simulink model "P3_Model_Final_V2"  (R2023b)
settings: Solver=VariableStepAuto  StartTime=0.0  StopTime=10.0  RelTol=1e-3
values from neighbouring files (symbols this model uses):
  DriveData = DriveData_urban    [Project3_RunSim_Final.m]
undefined symbols (not defined in the file or in its folder): batData, C0, C1, C2, carData, Iw, M, motorData, mph2mps, r, rps2rpm, Time
libraries: slpidlib x1
settings Model: Creator=jessi  LastModifiedBy=jessi

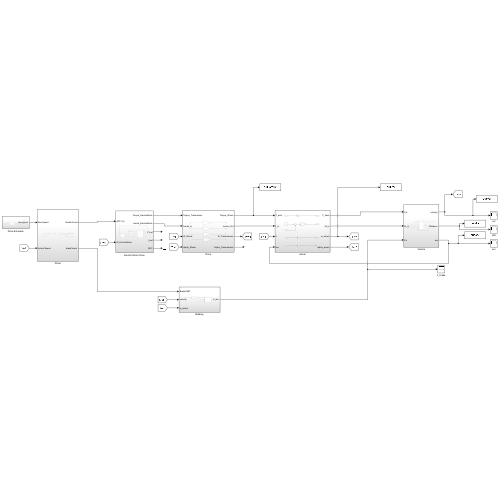
[thumbnail: Simulink's stored preview of the top-level diagram]
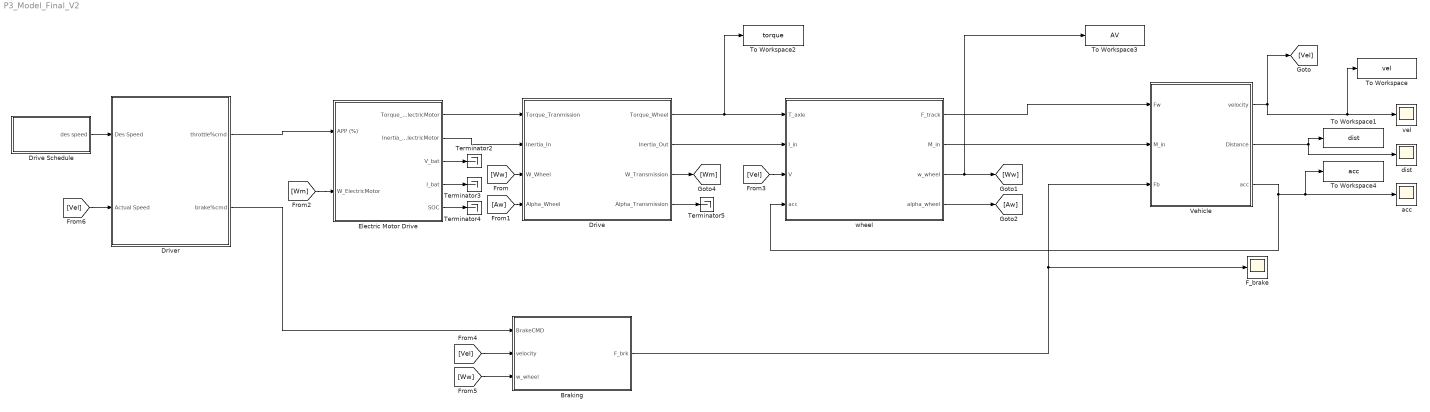
== system P3_Model_Final_V2 ==
  Braking : Subsystem
  Drive : Subsystem
  Drive Schedule : Subsystem
  "Driver " : Subsystem
  Electric Motor Drive : Subsystem
  F_brake : Scope
  Terminator{2..5} (4 alike) : Terminator
  To Workspace : ToWorkspace  VariableName=vel  SaveFormat=Timeseries  SampleTime=-1
  To Workspace1 : ToWorkspace  VariableName=dist  SaveFormat=Timeseries  SampleTime=-1
  To Workspace2 : ToWorkspace  VariableName=torque  SaveFormat=Timeseries  SampleTime=-1
  To Workspace3 : ToWorkspace  VariableName=AV  SaveFormat=Timeseries  SampleTime=-1
  To Workspace4 : ToWorkspace  VariableName=acc  SaveFormat=Timeseries  SampleTime=-1
  Vehicle : Subsystem
  acc : Scope
  dist : Scope
  vel : Scope
  "wheel " : Subsystem
  wires:
  [Ww] -> Braking/3(w_wheel)
  [Vel] -> Braking/2("velocity ")
  "wheel "/3(w_wheel) -> To Workspace3/1, [Ww]
  "wheel "/1(F_track) -> Vehicle/1("Fw ")
  [Wm] -> Electric Motor Drive/2(W_ElectricMotor)
  "wheel "/2(M_in) -> Vehicle/2("M_in ")
  [Ww] -> Drive/3(W_Wheel)
  Drive/1(Torque_Wheel) -> To Workspace2/1, "wheel "/1(T_axle)
  Drive/2(Inertia_Out) -> "wheel "/2(I_in)
  Electric Motor Drive/4(I_bat) -> Terminator3/1
  [Vel] -> "wheel "/3(V)
  Electric Motor Drive/5(SOC) -> Terminator4/1
  Electric Motor Drive/3(V_bat) -> Terminator2/1
  Vehicle/2("Distance ") -> dist/1, To Workspace1/1
  Braking/1("F_brk ") -> F_brake/1, Vehicle/3("Fb ")
  Drive/4(Alpha_Transmission) -> Terminator5/1
  Electric Motor Drive/2(Inertia_ElectricMotor) -> Drive/2(Inertia_In)
  Vehicle/3(acc) -> "wheel "/4(acc), To Workspace4/1, acc/1
  Vehicle/1("velocity ") -> To Workspace/1, vel/1, [Vel]
  Electric Motor Drive/1(Torque_ElectricMotor) -> Drive/1(Torque_Tranmission)
  "wheel "/4(alpha_wheel) -> [Aw]
  [Aw] -> Drive/4(Alpha_Wheel)
  Drive/3(W_Transmission) -> [Wm]
  Drive Schedule/1("des speed ") -> "Driver "/1("Des Speed ")
  [Vel] -> "Driver "/2(Actual Speed)
  "Driver "/1(throttle%cmd) -> Electric Motor Drive/1(APP (%))
  "Driver "/2("brake%cmd ") -> Braking/1("BrakeCMD ")

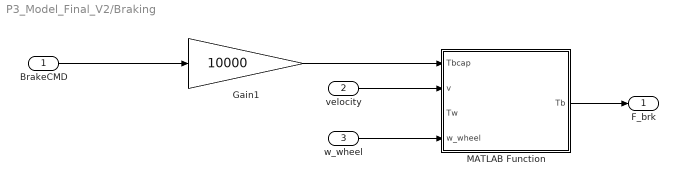
== system P3_Model_Final_V2/Braking ==
  "BrakeCMD " : Inport
  "velocity " : Inport  Port=2
  w_wheel : Inport  Port=3
  Gain1 : Gain  Gain=10000
  MATLAB Function : MATLAB Function  TreatAsAtomicUnit=on
  "F_brk " : Outport  VectorParamsAs1DForOutWhenUnconnected=off
  wires:
  "BrakeCMD "/1 -> Gain1/1
  Gain1/1 -> MATLAB Function/1(Tbcap)
  MATLAB Function/1(Tb) -> "F_brk "/1
  "velocity "/1 -> MATLAB Function/2(v)
  w_wheel/1 -> MATLAB Function/4(w_wheel)

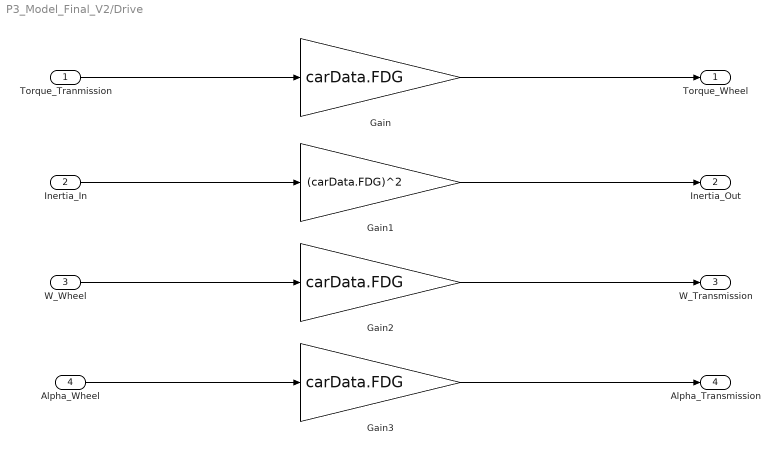
== system P3_Model_Final_V2/Drive ==
  Torque_Tranmission : Inport
  Inertia_In : Inport  Port=2
  W_Wheel : Inport  Port=3
  Alpha_Wheel : Inport  Port=4
  Gain : Gain  Gain=carData.FDG
  Gain1 : Gain  Gain=(carData.FDG)^2
  Gain2 : Gain  Gain=carData.FDG
  Gain3 : Gain  Gain=carData.FDG
  Torque_Wheel : Outport
  Inertia_Out : Outport  Port=2
  W_Transmission : Outport  Port=3
  Alpha_Transmission : Outport  Port=4
  wires:
  Torque_Tranmission/1 -> Gain/1
  Inertia_In/1 -> Gain1/1
  W_Wheel/1 -> Gain2/1
  Alpha_Wheel/1 -> Gain3/1
  Gain/1 -> Torque_Wheel/1
  Gain1/1 -> Inertia_Out/1
  Gain2/1 -> W_Transmission/1
  Gain3/1 -> Alpha_Transmission/1

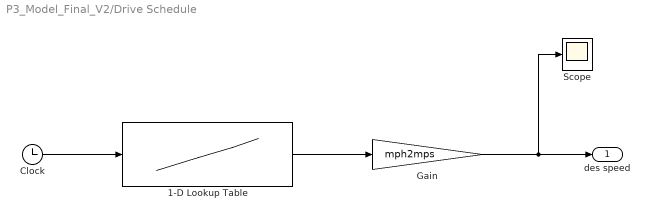
== system P3_Model_Final_V2/Drive Schedule ==
  1-D Lookup Table : Lookup_n-D  NumberOfTableDimensions=1  BreakpointsForDimension1=Time  Table=DriveData  InternalRulePriority=Speed  RndMeth=Simplest
  Clock : Clock
  Gain : Gain  Gain=mph2mps
  Scope : Scope
  "des speed " : Outport  VectorParamsAs1DForOutWhenUnconnected=off
  wires:
  Clock/1 -> 1-D Lookup Table/1
  1-D Lookup Table/1 -> Gain/1
  Gain/1 -> "des speed "/1, Scope/1

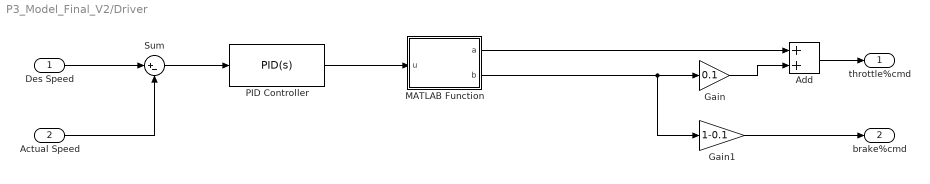
== system P3_Model_Final_V2/Driver  ==
  "Des Speed " : Inport
  Actual Speed : Inport  Port=2
  Add : Sum
  Gain : Gain  Gain=0.1
  Gain1 : Gain  Gain=1-0.1
  MATLAB Function : MATLAB Function  TreatAsAtomicUnit=on
  PID Controller : slpidlib/PID Controller  Controller=PID  Form=Parallel  TimeDomain=Continuous-time  UseExternalTs=off  SampleTime=-1  IntegratorMethod=Forward Euler  FilterMethod=Forward Euler  ControllerParametersSource=internal  P=0.55  I=0  UseKiTs=off  D=0  N=100  UseFilter=on  TunerSelectOption=Transfer Function Based (PID Tuner App)  InitialConditionSource=internal  InitialConditionForIntegrator=0  InitialConditionForFilter=0  DifferentiatorICPrevScaledInput=0  ExternalReset=none  TrackingMode=off  Kt=1  LimitOutput=on  SatLimitsSource=internal  UpperSaturationLimit=1  LowerSaturationLimit=-1  LinearizeAsGain=off  AntiWindupMode=none  Kb=1  LimitIntegrator=off  UpperIntegratorSaturationLimit=inf  LowerIntegratorSaturationLimit=-inf  POutMin=[]  POutMax=[]  IOutMin=[]  IOutMax=[]  DOutMin=[]  DOutMax=[]  NOutMin=[]  NOutMax=[]  SumOutMin=[]  SumOutMax=[]  SaturationOutMin=[]  SaturationOutMax=[]  PParamMin=[]  PParamMax=[]  IParamMin=[]  IParamMax=[]  DParamMin=[]  DParamMax=[]  NParamMin=[]  NParamMax=[]  KbParamMin=[]  KbParamMax=[]  KtParamMin=[]  KtParamMax=[]  KbOutMin=[]  KbOutMax=[]  KtOutMin=[]  KtOutMax=[]  IntegratorOutMin=[]  IntegratorOutMax=[]  FilterOutMin=[]  FilterOutMax=[]  SumI1OutMin=[]  SumI1OutMax=[]  SumI2OutMin=[]  SumI2OutMax=[]  SumI3OutMin=[]  SumI3OutMax=[]  SumI4OutMin=[]  SumI4OutMax=[]  SumDOutMin=[]  SumDOutMax=[]  DifferentiatorOutMin=[]  DifferentiatorOutMax=[]  FilterDiffOutCoefMin=[]  FilterDiffOutCoefMax=[]  ReciprocalOutMin=[]  ReciprocalOutMax=[]  SumDenOutMin=[]  SumDenOutMax=[]  SumNumOutMin=[]  SumNumOutMax=[]  DivideOutMin=[]  DivideOutMax=[]  UdiffTsProdOutMin=[]  UdiffTsProdOutMax=[]  NTsProdOutMin=[]  NTsProdOutMax=[]  UintegralTsProdOutMin=[]  UintegralTsProdOutMax=[]  UngainTsProdOutMin=[]  UngainTsProdOutMax=[]  ClampingZeroOutDataTypeStr=Inherit: Inherit via back propagation  ClampingZeroOutMin=[]  ClampingZeroOutMax=[]  FilterDenConstantOutDataTypeStr=Inherit: Inherit via back propagation  FilterDenConstantOutMin=[]  FilterDenConstantOutMax=[]  PCopyOutDataTypeStr=Inherit: Inherit via back propagation  PCopyOutMin=[]  PCopyOutMax=[]  NCopyOutDataTypeStr=Inherit: Inherit via back propagation  NCopyOutMin=[]  NCopyOutMax=[]  IntegratorContinuousStateAttributes=''  IntegratorStateMustResolveToSignalObject=off  IntegratorRTWStateStorageClass=Auto  FilterContinuousStateAttributes=''  FilterStateMustResolveToSignalObject=off  FilterRTWStateStorageClass=Auto  ParallelPVariant=InternalParameters  IdealPVariant=Disabled  IVariant=InternalParameters  DVariant=InternalParameters  IntegratorVariant=Continuous  SatVariant=Enabled  AWVariant=Passthrough  PCopyVariant=Disabled  TRVariant=Disabled  FdbkBlocksVariant=Forward  IdealPFdbkVariant=Disabled  SatFdbkVariant=Disabled  DerivativeFilterVariant=ContFilter  NVariant=InternalParameters  NCopyVariant=Disabled  FilterICVariant=InternalICsFilter  IntegratorICVariant=InternalICs  ExternalResetVariant=Disabled  TRSumVariant=Passthrough  SumFdbkVariant=Disabled  SumVariant=Sum_PID  TsampFilterVariant=InternalTs  TsampNgainVariant=Passthrough  TsampIntegralVariant=Disabled_SignalSpec  ExternalSaturationOutDataTypeStr=Inherit: Same as second input
  Sum : Sum  Inputs=|+-
  throttle%cmd : Outport
  "brake%cmd " : Outport  Port=2
  wires:
  MATLAB Function/1(a) -> Add/1
  Gain/1 -> Add/2
  Add/1 -> throttle%cmd/1
  Gain1/1 -> "brake%cmd "/1
  MATLAB Function/2(b) -> Gain1/1, Gain/1
  Sum/1 -> PID Controller/1
  PID Controller/1 -> MATLAB Function/1(u)
  "Des Speed "/1 -> Sum/1
  Actual Speed/1 -> Sum/2

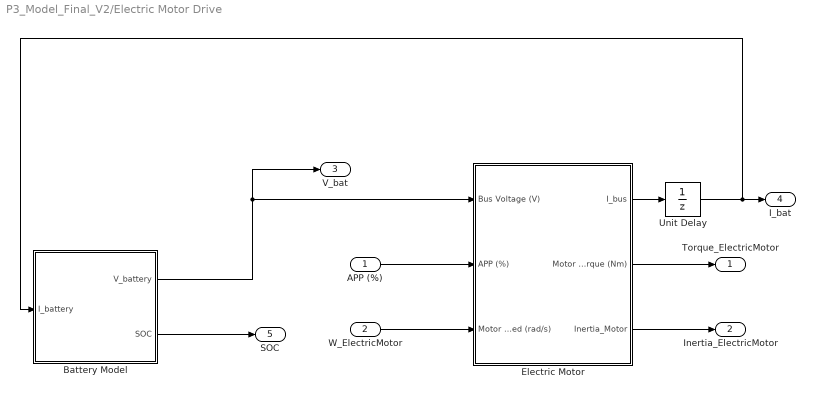
== system P3_Model_Final_V2/Electric Motor Drive ==
  APP (%) : Inport
  W_ElectricMotor : Inport  Port=2
  Battery Model : Subsystem  TreatAsAtomicUnit=on
  Electric Motor : Subsystem  TreatAsAtomicUnit=on
  Unit Delay : UnitDelay  SampleTime=-1  HasFrameUpgradeWarning=on
  Torque_ElectricMotor : Outport
  Inertia_ElectricMotor : Outport  Port=2
  V_bat : Outport  Port=3
  I_bat : Outport  Port=4
  SOC : Outport  Port=5
  wires:
  Electric Motor/2(Motor Torque (Nm)) -> Torque_ElectricMotor/1
  Battery Model/2(SOC) -> SOC/1
  Electric Motor/3(Inertia_Motor) -> Inertia_ElectricMotor/1
  W_ElectricMotor/1 -> Electric Motor/3(Motor Speed (rad/s))
  Electric Motor/1(I_bus) -> Unit Delay/1
  APP (%)/1 -> Electric Motor/2(APP (%))
  Battery Model/1(V_battery) -> Electric Motor/1(Bus Voltage (V)), V_bat/1
  Unit Delay/1 -> Battery Model/1(I_battery), I_bat/1

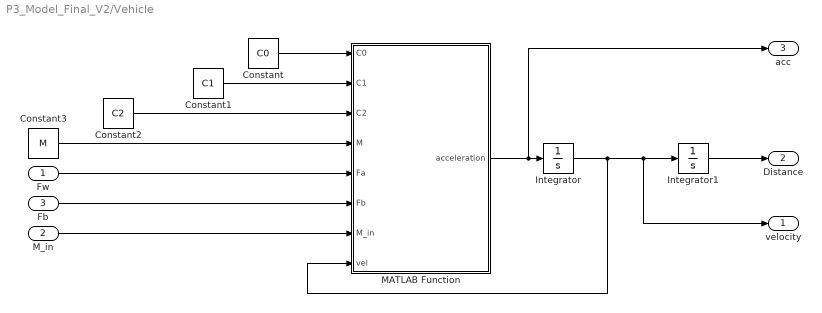
== system P3_Model_Final_V2/Vehicle ==
  "Fw " : Inport
  "M_in " : Inport  Port=2
  "Fb " : Inport  Port=3
  Constant : Constant  Value=C0
  Constant1 : Constant  Value=C1
  Constant2 : Constant  Value=C2
  Constant3 : Constant  Value=M
  Integrator : Integrator  LimitOutput=on  LowerSaturationLimit=0
  Integrator1 : Integrator
  MATLAB Function : MATLAB Function  TreatAsAtomicUnit=on
  "velocity " : Outport  VectorParamsAs1DForOutWhenUnconnected=off
  "Distance " : Outport  Port=2  VectorParamsAs1DForOutWhenUnconnected=off
  acc : Outport  Port=3
  wires:
  Constant1/1 -> MATLAB Function/2(C1)
  Constant/1 -> MATLAB Function/1(C0)
  MATLAB Function/1(acceleration) -> acc/1, Integrator/1
  Constant2/1 -> MATLAB Function/3(C2)
  Constant3/1 -> MATLAB Function/4(M)
  "Fw "/1 -> MATLAB Function/5(Fa)
  "Fb "/1 -> MATLAB Function/6(Fb)
  Integrator/1 -> MATLAB Function/8(vel), "velocity "/1, Integrator1/1
  Integrator1/1 -> "Distance "/1
  "M_in "/1 -> MATLAB Function/7(M_in)

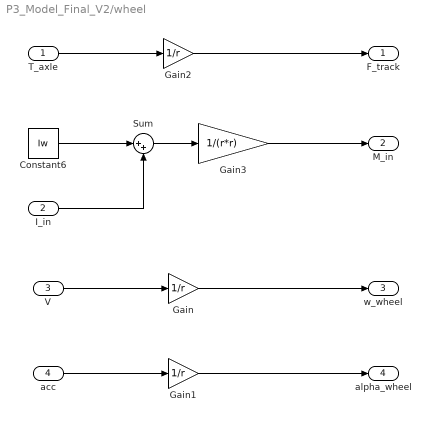
== system P3_Model_Final_V2/wheel  ==
  T_axle : Inport
  I_in : Inport  Port=2
  V : Inport  Port=3
  acc : Inport  Port=4
  Constant6 : Constant  Value=Iw
  Gain : Gain  Gain=1/r
  Gain1 : Gain  Gain=1/r
  Gain2 : Gain  Gain=1/r
  Gain3 : Gain  Gain=1/(r*r)
  Sum : Sum  Inputs=|++
  F_track : Outport
  M_in : Outport  Port=2
  w_wheel : Outport  Port=3
  alpha_wheel : Outport  Port=4
  wires:
  Gain/1 -> w_wheel/1
  V/1 -> Gain/1
  acc/1 -> Gain1/1
  Gain1/1 -> alpha_wheel/1
  T_axle/1 -> Gain2/1
  Gain2/1 -> F_track/1
  Gain3/1 -> M_in/1
  Constant6/1 -> Sum/1
  I_in/1 -> Sum/2
  Sum/1 -> Gain3/1

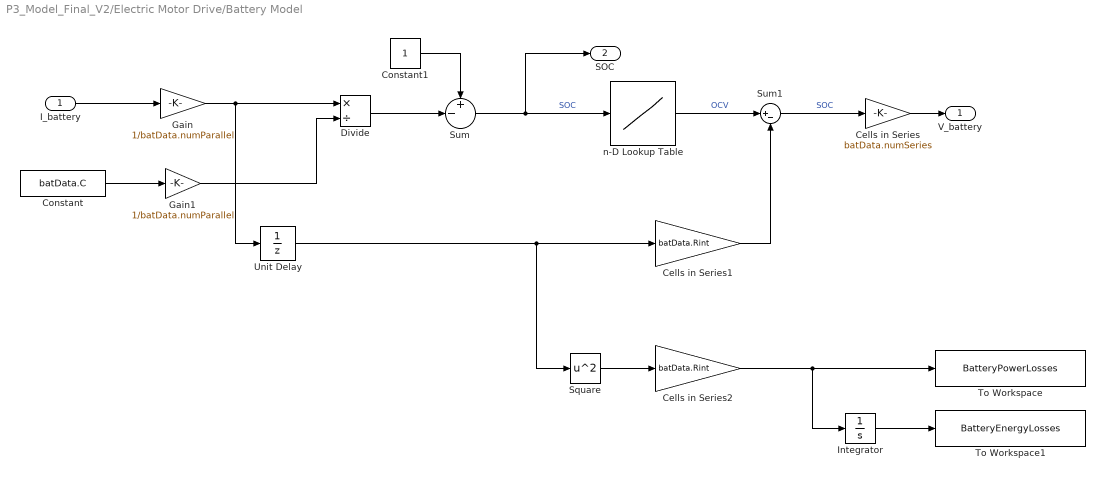
== system P3_Model_Final_V2/Electric Motor Drive/Battery Model ==
  I_battery : Inport
  Cells in Series : Gain  Gain=batData.numSeries
  Cells in Series1 : Gain  Gain=batData.Rint
  Cells in Series2 : Gain  Gain=batData.Rint
  Constant : Constant  Value=batData.C
  Constant1 : Constant
  Divide : Product  Inputs=*/
  Gain : Gain  Gain=1/batData.numParallel
  Gain1 : Gain  Gain=1/batData.numParallel
  Integrator : Integrator
  Square : Math  Operator=square
  Sum : Sum  Inputs=+-|
  Sum1 : Sum  Inputs=|+-
  To Workspace : ToWorkspace  VariableName=BatteryPowerLosses  SaveFormat=Timeseries  SampleTime=-1
  To Workspace1 : ToWorkspace  VariableName=BatteryEnergyLosses  SaveFormat=Timeseries  SampleTime=-1
  Unit Delay : UnitDelay  SampleTime=-1  HasFrameUpgradeWarning=on
  n-D Lookup Table : Lookup_n-D  NumberOfTableDimensions=1  BreakpointsForDimension1=batData.SOC  BreakpointsForDimension3=[5, 7]  Table=batData.OCV  InternalRulePriority=Speed  RndMeth=Simplest
  V_battery : Outport
  SOC : Outport  Port=2
  wires:
  I_battery/1 -> Gain/1
  Gain/1 -> Unit Delay/1, Divide/1
  Gain1/1 -> Divide/2
  Constant/1 -> Gain1/1
  Constant1/1 -> Sum/1
  Divide/1 -> Sum/2
  Sum/1 -> SOC/1, n-D Lookup Table/1  "SOC"
  n-D Lookup Table/1 -> Sum1/1  "OCV"
  Cells in Series/1 -> V_battery/1
  Sum1/1 -> Cells in Series/1  "SOC"
  Cells in Series1/1 -> Sum1/2
  Square/1 -> Cells in Series2/1
  Cells in Series2/1 -> Integrator/1, To Workspace/1
  Integrator/1 -> To Workspace1/1
  Unit Delay/1 -> Square/1, Cells in Series1/1

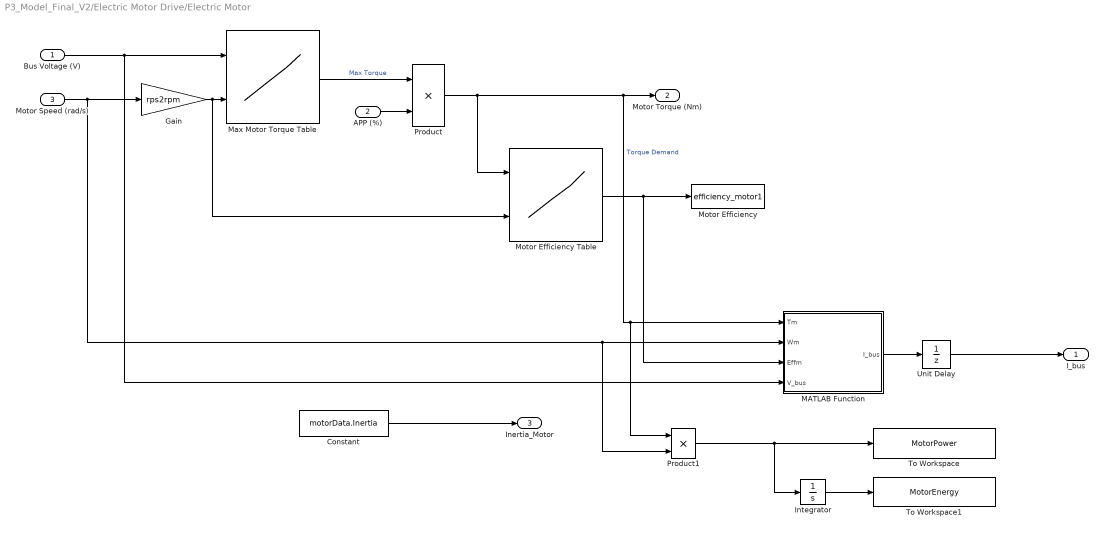
== system P3_Model_Final_V2/Electric Motor Drive/Electric Motor ==
  Bus Voltage (V) : Inport
  APP (%) : Inport  Port=2
  Motor Speed (rad/s) : Inport  Port=3
  Constant : Constant  Value=motorData.Inertia
  Gain : Gain  Gain=rps2rpm
  Integrator : Integrator
  MATLAB Function : MATLAB Function  TreatAsAtomicUnit=on
  Max Motor Torque Table : Lookup_n-D  BreakpointsForDimension1=motorData.vbus  BreakpointsForDimension2=motorData.rpm  BreakpointsForDimension3=[5, 7]  Table=motorData.maxtorque  InternalRulePriority=Speed  RndMeth=Simplest
      settings: InputPortMap=u0,u1
  Motor Efficiency : ToWorkspace  VariableName=efficiency_motor1  SaveFormat=Timeseries  SampleTime=-1
  Motor Efficiency Table : Lookup_n-D  BreakpointsForDimension1=motorData.eta_torque  BreakpointsForDimension2=motorData.eta_speed  BreakpointsForDimension3=[5, 7]  Table=motorData.eta_val  InternalRulePriority=Speed  RndMeth=Simplest
      settings: InputPortMap=u0,u1
  Product : Product
  Product1 : Product
  To Workspace : ToWorkspace  VariableName=MotorPower  SaveFormat=Timeseries  SampleTime=-1
  To Workspace1 : ToWorkspace  VariableName=MotorEnergy  SaveFormat=Timeseries  SampleTime=-1
  Unit Delay : UnitDelay  SampleTime=-1  HasFrameUpgradeWarning=on
  I_bus : Outport
  Motor Torque (Nm) : Outport  Port=2
  Inertia_Motor : Outport  Port=3
  wires:
  Constant/1 -> Inertia_Motor/1
  APP (%)/1 -> Product/2
  Max Motor Torque Table/1 -> Product/1  "Max Torque"
  Product/1 -> Motor Efficiency Table/1, Product1/1, MATLAB Function/1(Tm), Motor Torque (Nm)/1  "Torque Demand"
  Gain/1 -> Motor Efficiency Table/2, Max Motor Torque Table/2
  Motor Speed (rad/s)/1 -> Gain/1, Product1/2, MATLAB Function/2(Wm)
  Motor Efficiency Table/1 -> MATLAB Function/3(Effm), Motor Efficiency/1
  Integrator/1 -> To Workspace1/1
  Product1/1 -> Integrator/1, To Workspace/1
  MATLAB Function/1(I_bus) -> Unit Delay/1
  Unit Delay/1 -> I_bus/1
  Bus Voltage (V)/1 -> MATLAB Function/4(V_bus), Max Motor Torque Table/1

== matlab function P3_Model_Final_V2/Driver /MATLAB Function ==
  data: u input; a output; b output
% Checks if there is a difference between actual speed and desired speed

% u is calculated using the sum function in the simulink model

function [a,b] = fcn(u)

if u>0 % If the difference is greater than zero, then we need to speed up since actual speed is less than desired speed
    acc=u; % We send how much we need to speed up to the throttle command
    brk=0; % Do nothing for the break command
elseif u<0 % If the difference is less than zero, then we need to slow down since the actual speed is less than the desired speed
    acc=0; % Do nothing for throttle command
    brk=-u; % We send how much we need to break to the break command
else % If the desired and actual speed is the same
    acc=0; % Do nothing for throttle command
    brk=0; % Do nothing for the break command
end
a= acc; % storing how much acceleration required to a
b= brk; % storing how much break acceleration required to b

== matlab function P3_Model_Final_V2/Vehicle/MATLAB Function ==
  data: C0 input; acceleration output; C1 input; C2 input; M input; Fa input; Fb input; M_in input; vel input
function acceleration   = vehicle(C0,C1,C2,M,Fa,Fb,M_in, vel)

acceleration = (((Fa-Fb))-(C0+ C1*vel + C2*(vel)^2))/(M+M_in);


% Fa: Force from wheel.
% Fb: Force from brake.
% -(C0+ C1*vel + C2*(vel)^2)): Force from drag (opposite direction of motion)

== matlab function P3_Model_Final_V2/Electric Motor Drive/Electric Motor/MATLAB Function ==
  data: Tm input; I_bus output; Wm input; Effm input; V_bus input
function I_bus = fcn(Tm,Wm,Effm,V_bus)

%I_bus = (Tm*Wm/Effm)/V_bus;

Pm=Tm*Wm;
sgnPm = Pm/(abs(Pm)+0.001);
I_bus = ( (Pm) * (Effm)^(sgnPm) ) / V_bus;

== matlab function P3_Model_Final_V2/Braking/MATLAB Function ==
  data: Tbcap input; Tb output; v input; Tw input; w_wheel input
function Tb = fcn(Tbcap, v, Tw,w_wheel)
Tb = Tbcap * v/(abs(v)+0.001);
end

% wrong, more logic needs to be added to this
% try to find where to incorporate Tw and w_wheel into function
